simulink model "ControlBooleC1P1"  (R2022b)
settings: Solver=ode45  StartTime=0.0  StopTime=10  RelTol=1e-7  AbsTol=1e-7  EnableMultiTasking=on
settings Model: Creator=Helbert  LastModifiedBy=rogaj
settings SolverCC: AutoScaleAbsTol=off  ZeroCrossControl=DisableAll  AlgebraicLoopSolver=TrustRegion
settings DataIOCC: LimitDataPoints=on  SaveFormat=Array  SignalLoggingSaveFormat=ModelDataLogs  ReturnWorkspaceOutputs=off
settings OptimizationCC: InitFltsAndDblsToZero=on  LifeSpan=inf
settings DebuggingCC: SaveWithParameterizedLinksMsg=none  UnderspecifiedInitializationDetection=Classic  MergeDetectMultiDrivingBlocksExec=none  SignalResolutionControl=TryResolveAllWithWarning  SolverPrmCheckMsg=warning  MultiTaskDSMMsg=warning  MultiTaskCondExecSysMsg=none  UnconnectedInputMsg=warning  UnconnectedOutputMsg=warning  UnconnectedLineMsg=warning  SFUnexpectedBacktrackingDiag=warning  SFNoUnconditionalDefaultTransitionDiag=warning  SFExecutionAtInitializationDiag=none  SFMachineParentedDataDiag=warning  ArithmeticOperatorsInVariantConditions=warning
settings HardwareCC: ProdBitPerPointer=32  ProdBitPerSizeT=32  ProdBitPerPtrDiffT=32  ProdLargestAtomicFloat=None  ProdIntDivRoundTo=Undefined  ProdEndianess=Unspecified  ProdWordSize=32  ProdHWDeviceType=32-bit Generic
settings ModelReferenceCC: EnableRefExpFcnMdlSchedulingChecks=on  PropagateSignalLabelsOutOfModel=off
settings SFSimCC: SimUseLocalCustomCode=off  CustomCodeUndefinedFunction=UseInterfaceOnly
settings RTWCC: RTWUseLocalCustomCode=off
settings CodeAppCC: StateflowObjectComments=on
settings GRTTargetCC: TargetFcnLib=ansi_tfl_tmw.mat  TargetLangStandard=C89/C90 (ANSI)  CombineOutputUpdateFcns=off  GRTInterface=on
settings ConfigComp: CovMetricSettings=dw  CovSaveCumulativeToWorkspaceVar=on  CovSaveSingleToWorkspaceVar=on  CovExternalEMLEnable=off

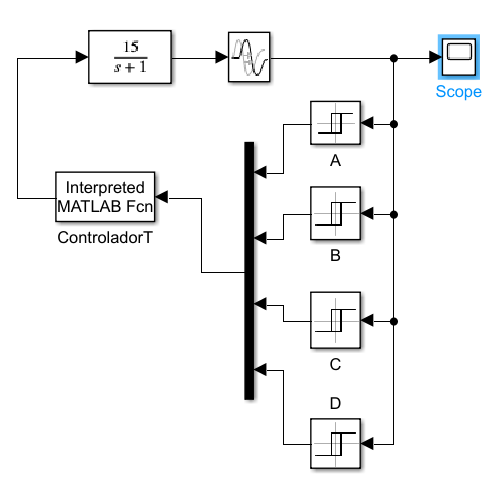
[thumbnail: Simulink's stored preview of the top-level diagram]
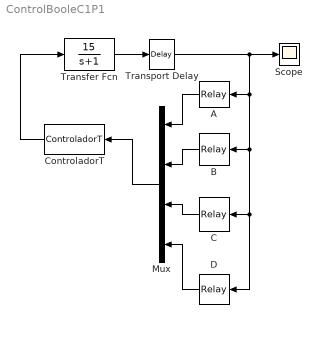
== system ControlBooleC1P1 ==
  A : Relay  OnSwitchValue=4  OffSwitchValue=4
  B : Relay  OnSwitchValue=3  OffSwitchValue=2
  C : Relay  OnSwitchValue=2  OffSwitchValue=1
  ControladorT : MATLABFcn  MATLABFcn=ControladorT
  D : Relay  Tag=D  Description=D  OnSwitchValue=1  OffSwitchValue=0
  Mux : Mux
  Scope : Scope
  Transfer Fcn : TransferFcn  Numerator=[15]  Denominator=[1 1]
  Transport Delay : TransportDelay  DelayTime=0.5
  wires:
  Transfer Fcn/1 -> Transport Delay/1
  A/1 -> Mux/1
  B/1 -> Mux/2
  C/1 -> Mux/3
  Mux/1 -> ControladorT/1
  ControladorT/1 -> Transfer Fcn/1
  D/1 -> Mux/4
  Transport Delay/1 -> D/1, C/1, B/1, A/1, Scope/1
